simulink model "DC_Microgrid_Complete"  (R2022a)
settings: Solver=ode4  StartTime=0.0  StopTime=86400  FixedStep=1  RelTol=1e-3
settings Model: Creator=nivas  LastModifiedBy=nivas

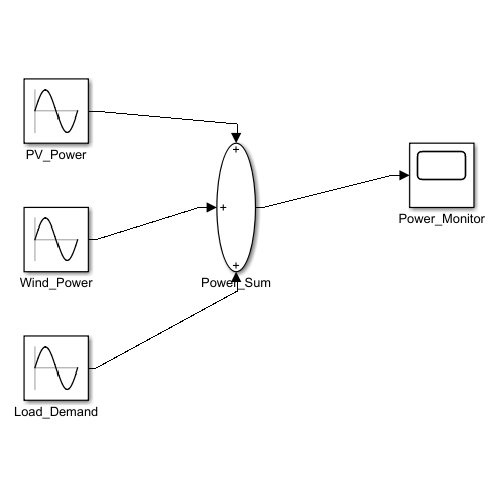
[thumbnail: Simulink's stored preview of the top-level diagram]
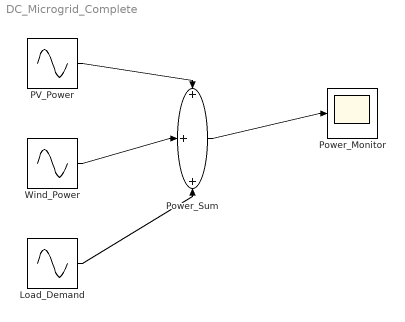
== system DC_Microgrid_Complete ==
  Load_Demand : Sin  Amplitude=35000  Bias=35000  Frequency=1/43200  SampleTime=0
  PV_Power : Sin  Amplitude=50000  Bias=30000  Frequency=1/86400  SampleTime=0
  Power_Monitor : Scope
  Power_Sum : Sum  Inputs=+++
  Wind_Power : Sin  Amplitude=15000  Bias=20000  Frequency=2/86400  SampleTime=0
  wires:
  PV_Power/1 -> Power_Sum/1
  Wind_Power/1 -> Power_Sum/2
  Load_Demand/1 -> Power_Sum/3
  Power_Sum/1 -> Power_Monitor/1
